simulink model "pl4_p"  (R2017b)
settings: Solver=VariableStepAuto  StartTime=0.0  StopTime=4  RelTol=1e-3
values from neighbouring files (symbols this model uses):
  a = m*r*r*Rm + Kg*Kg*Jm*Rm    (= 0.0001128156198)    [Lab4.m]    (also in Prelab4.m)
  b = Kg*Kg*Kt*Km    (= 0.00080972686249)    [Lab4.m]    (also in Prelab4.m)
  c = Kg*Kt*r    (= 0.000180978252)    [Lab4.m]    (also in Prelab4.m)
  K = 36.07    [Lab4.m]    (also in Prelab4.m = 15)
settings Model: Creator=Jenny  LastModifiedBy=Jenny

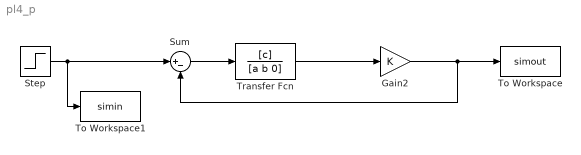
== system pl4_p ==
  Gain2 : Gain  Gain=K
  Step : Step  Time=0  After=0.15  SampleTime=0
  Sum : Sum  Inputs=|+-
  To Workspace : ToWorkspace  VariableName=simout  SaveFormat=Timeseries  SampleTime=-1
  To Workspace1 : ToWorkspace  VariableName=simin  SaveFormat=Timeseries  SampleTime=-1
  Transfer Fcn : TransferFcn  Numerator=[c]  Denominator=[a b 0]
  wires:
  Step/1 -> Sum/1, To Workspace1/1
  Sum/1 -> Transfer Fcn/1
  Transfer Fcn/1 -> Gain2/1
  Gain2/1 -> Sum/2, To Workspace/1
